simulink model "F104_Project_NEw_Aero_final_replacing"  (R2013a)
settings: Solver=ode45  StartTime=0.0  StopTime=50  FixedStep=0.01  RelTol=0.01
values from neighbouring files (symbols this model uses):
  b_w = 21.94    [Donee.m]
  C = 9.55    [Donee.m]
  Cl_beta = -0.09    [CX.m]    (also in CY.m; CZ.m; Cm.m; Cn.m)
  Cl_delta_aileron = 0.017    [Donee.m]
  CL_delta_elevator = 0.52    [Donee.m]
  Cl_delta_rudder = 0.008    [Donee.m]
  Cm_alpha = CL_alpha*CmoCL    [Aerodynamic_Dervatives.m]
  Cm_alpha_dot = - CL_alpha_dot * (l_t/C)    [Aerodynamic_Dervatives.m]
  Cm_delta_elevator = -0.2    [Donee.m]
  Cm_q = - CL_q * (l_t/C)    [Aerodynamic_Dervatives.m]
  Cm_u = 0    [Aerodynamic_Dervatives.m]
  Cn_beta = 0.0024    [Aerodynamic_Dervatives.m]    (also in CX.m = 0.24; CY.m = 0.24; CZ.m = 0.24; Cm.m = 0.24)
  Cn_delta_aileron = 0.0025    [Donee.m]
  Cn_delta_rudder = -0.04    [Donee.m]
  CX_q = -CD_q    (= 0)    [Aerodynamic_Dervatives.m]
  Cy_delta_rudder = 0.05    [Donee.m]
  CZ_alpha_dot = - CL_alpha_dot    [Aerodynamic_Dervatives.m]
  CZ_q = -CL_q    [Aerodynamic_Dervatives.m]
  S_w = (Cr_w + Ct_w)*b_w/4    (= 95.762615)    [Donee.m]
undefined symbols (not defined in the file or in its folder): Cl_beta_dot, Cl_p, Cl_r, Cn_beta_dot, Cn_p, Cn_r, CX_alpha, CX_u, Cy_beta, Cy_beta_dot, Cy_r, CZ_alpha, CZ_u, ft, kg, lbm, m, s
libraries: aerolibconvert2 x6, aerolibasang x2, aerolib6dof2 x1, aerolibatmos2 x1
settings Model: Creator=Ibrahim_B92  LastModifiedBy=Ibrahim_B92

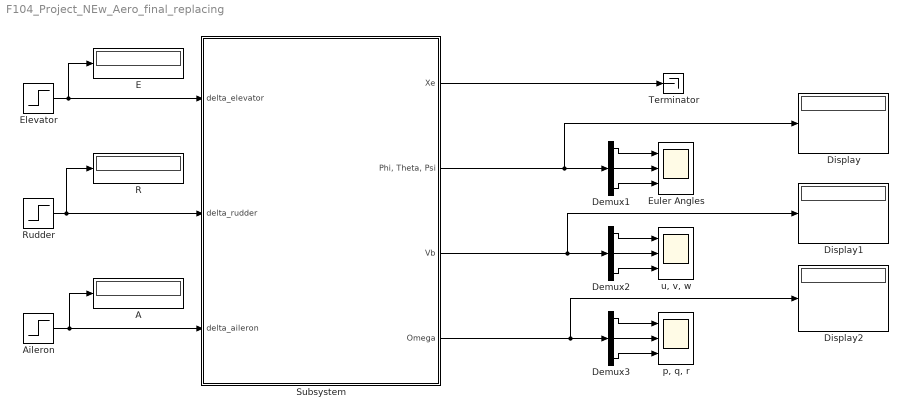
== system F104_Project_NEw_Aero_final_replacing ==
  A : Display
  Aileron : Step  Time=0  After=0  SampleTime=0
  Demux1 : Demux  Outputs=3
  Demux2 : Demux  Outputs=3
  Demux3 : Demux  Outputs=3
  Display : Display
  Display1 : Display
  Display2 : Display
  E : Display
  Elevator : Step  Time=0  After=0  SampleTime=0
  Euler Angles : Scope  NumInputPorts=3
      settings: TimeRange=16  YMin=0~-2~-5  YMax=1000~2~10
  R : Display
  Rudder : Step  Time=0  After=0  SampleTime=0
  Subsystem : Subsystem
  Terminator : Terminator
  "p, q, r" : Scope  NumInputPorts=3
      settings: TimeRange=10  YMin=-5~-5~-5  YMax=5~5~5  SaveName=ScopeData3
  "u, v, w" : Scope  NumInputPorts=3
      settings: TickLabels=on  TimeRange=16  YMin=-1000~-2000~-2000  YMax=2000~2000~2000  SaveName=ScopeData2
  wires:
  Subsystem/1(Xe) -> Terminator/1
  Demux1/1 -> Euler Angles/1
  Demux1/2 -> Euler Angles/2
  Demux1/3 -> Euler Angles/3
  Subsystem/2("Phi, Theta, Psi") -> Display/1, Demux1/1
  Demux2/1 -> "u, v, w"/1
  Demux2/2 -> "u, v, w"/2
  Demux2/3 -> "u, v, w"/3
  Subsystem/3(Vb) -> Display1/1, Demux2/1
  Demux3/1 -> "p, q, r"/1
  Demux3/2 -> "p, q, r"/2
  Demux3/3 -> "p, q, r"/3
  Subsystem/4(Omega) -> Display2/1, Demux3/1
  Rudder/1 -> Subsystem/2(delta_rudder), R/1
  Aileron/1 -> Subsystem/3(delta_aileron), A/1
  Elevator/1 -> Subsystem/1(delta_elevator), E/1

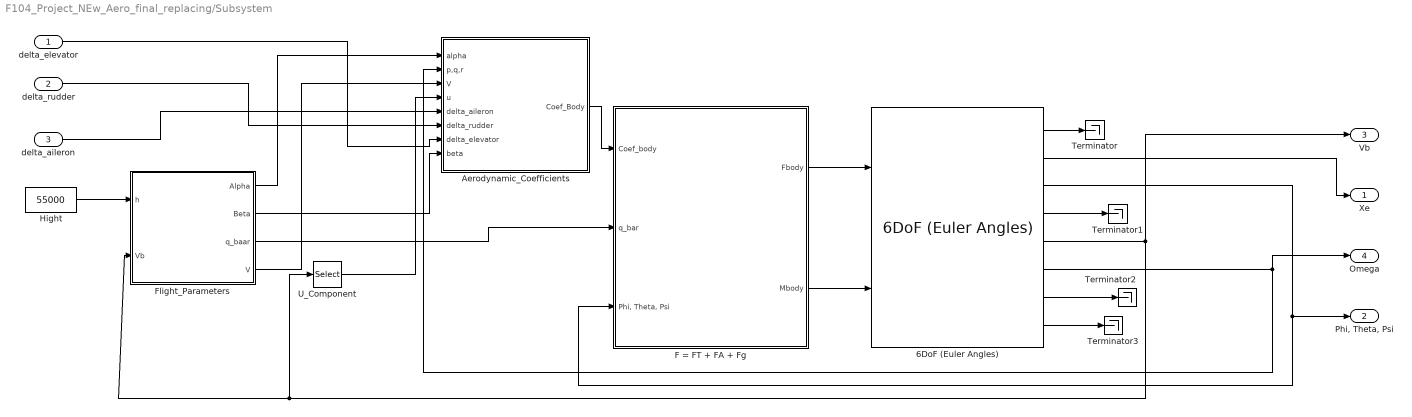
== system F104_Project_NEw_Aero_final_replacing/Subsystem ==
  delta_elevator : Inport
  delta_rudder : Inport  Port=2
  delta_aileron : Inport  Port=3
  6DoF (Euler Angles) : aerolib6dof2/6DoF (Euler Angles)  units=Metric (MKS)  mtype=Fixed  rep=Euler Angles  xme_0=|  Vm_0=|  eul_0=[0 0 0]  pm_0=[0 0 0]  mass_0=16300  mass_e=0.5  mass_f=2.0  inertia=Q  inertia_e=eye(3)  inertia_f=2*eye(3)  k_quat=1.0
      xme_0=|
      | [0
      | 0
      | -55000]
      Vm_0=|
      | [968*1.8
      | 0
      | 0]
  Aerodynamic_Coefficients : Subsystem
  F = FT + FA + Fg : Subsystem
  Flight_Parameters : Subsystem
  Hight : Constant  Value=55000
  Terminator{,1..3} (4 alike) : Terminator
  U_Component : Selector  InputPortWidth=3  IndexOptions=Index vector (dialog)  Indices=[1]  OutputSizes=1
  Xe : Outport
  "Phi, Theta, Psi" : Outport  Port=2
  Vb : Outport  Port=3
  Omega : Outport  Port=4
  wires:
  6DoF (Euler Angles)/2 -> Xe/1
  6DoF (Euler Angles)/3 -> F = FT + FA + Fg/3("Phi, Theta, Psi"), "Phi, Theta, Psi"/1
  6DoF (Euler Angles)/5 -> Flight_Parameters/2(Vb), U_Component/1, Vb/1
  6DoF (Euler Angles)/6 -> Aerodynamic_Coefficients/2(p,q,r), Omega/1
  F = FT + FA + Fg/1(Fbody) -> 6DoF (Euler Angles)/1
  F = FT + FA + Fg/2(Mbody) -> 6DoF (Euler Angles)/2
  Flight_Parameters/3(q_baar) -> F = FT + FA + Fg/2(q_bar)
  Flight_Parameters/1(Alpha) -> Aerodynamic_Coefficients/1(alpha)
  Flight_Parameters/2(Beta) -> Aerodynamic_Coefficients/8(beta)
  Hight/1 -> Flight_Parameters/1(h)
  Flight_Parameters/4(V) -> Aerodynamic_Coefficients/3(V)
  delta_elevator/1 -> Aerodynamic_Coefficients/7(delta_elevator)
  delta_rudder/1 -> Aerodynamic_Coefficients/6(delta_rudder)
  6DoF (Euler Angles)/1 -> Terminator/1
  6DoF (Euler Angles)/4 -> Terminator1/1
  6DoF (Euler Angles)/7 -> Terminator2/1
  6DoF (Euler Angles)/8 -> Terminator3/1
  U_Component/1 -> Aerodynamic_Coefficients/4(u)
  Aerodynamic_Coefficients/1(Coef_Body) -> F = FT + FA + Fg/1(Coef_body)
  delta_aileron/1 -> Aerodynamic_Coefficients/5(delta_aileron)

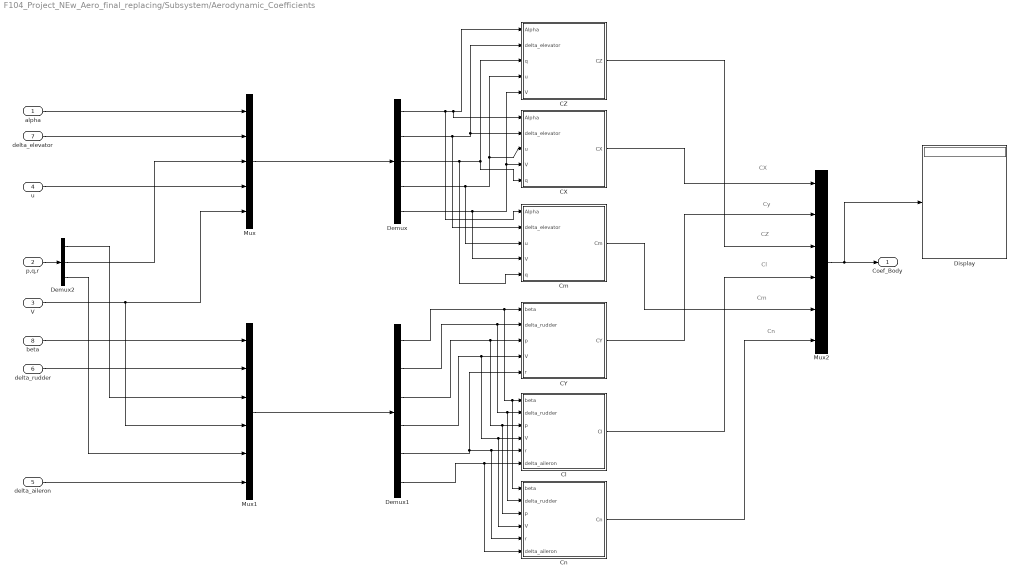
== system F104_Project_NEw_Aero_final_replacing/Subsystem/Aerodynamic_Coefficients ==
  note: Cn
  note: Cm
  note: Cl
  note: CZ
  note: Cy
  note: CX
  alpha : Inport
  p,q,r : Inport  Port=2
  V : Inport  Port=3
  u : Inport  Port=4
  delta_aileron : Inport  Port=5
  delta_rudder : Inport  Port=6
  delta_elevator : Inport  Port=7
  beta : Inport  Port=8
  CX : Subsystem
  CY : Subsystem
  CZ : Subsystem
  Cl : Subsystem
  Cm : Subsystem
  Cn : Subsystem
  Demux : Demux  Outputs=5
  Demux1 : Demux  Outputs=6
  Demux2 : Demux  Outputs=3
  Display : Display
  Mux : Mux  Inputs=5
  Mux1 : Mux  Inputs=6
  Mux2 : Mux  Inputs=6
  Coef_Body : Outport
  wires:
  Demux/1 -> Cm/1(Alpha), CX/1(Alpha), CZ/1(Alpha)
  Demux/2 -> Cm/2(delta_elevator), CX/2(delta_elevator), CZ/2(delta_elevator)
  Demux/3 -> Cm/5(q), CZ/3(q), CX/5(q)
  Demux/5 -> Cm/4(V), CX/4(V), CZ/5(V)
  Demux/4 -> Cm/3(u), CX/3(u), CZ/4(u)
  Demux1/1 -> Cn/1(beta), Cl/1(beta), CY/1(beta)
  Demux1/2 -> Cn/2(delta_rudder), Cl/2(delta_rudder), CY/2(delta_rudder)
  Demux1/4 -> Cn/4(V), Cl/4(V), CY/4(V)
  Demux1/5 -> CY/5(r), Cl/5(r), Cn/5(r)
  Demux1/6 -> Cn/6(delta_aileron), Cl/6(delta_aileron)
  Demux1/3 -> Cl/3(p), Cn/3(p), CY/3(p)
  Mux/1 -> Demux/1
  alpha/1 -> Mux/1
  p,q,r/1 -> Demux2/1
  delta_elevator/1 -> Mux/2
  Demux2/2 -> Mux/3
  u/1 -> Mux/4
  V/1 -> Mux1/4, Mux/5
  Mux1/1 -> Demux1/1
  beta/1 -> Mux1/1
  delta_rudder/1 -> Mux1/2
  Demux2/1 -> Mux1/3
  Demux2/3 -> Mux1/5
  delta_aileron/1 -> Mux1/6
  CX/1(CX) -> Mux2/1
  CY/1(CY) -> Mux2/2
  CZ/1(CZ) -> Mux2/3
  Cl/1(Cl) -> Mux2/4
  Cm/1(Cm) -> Mux2/5
  Cn/1(Cn) -> Mux2/6
  Mux2/1 -> Display/1, Coef_Body/1

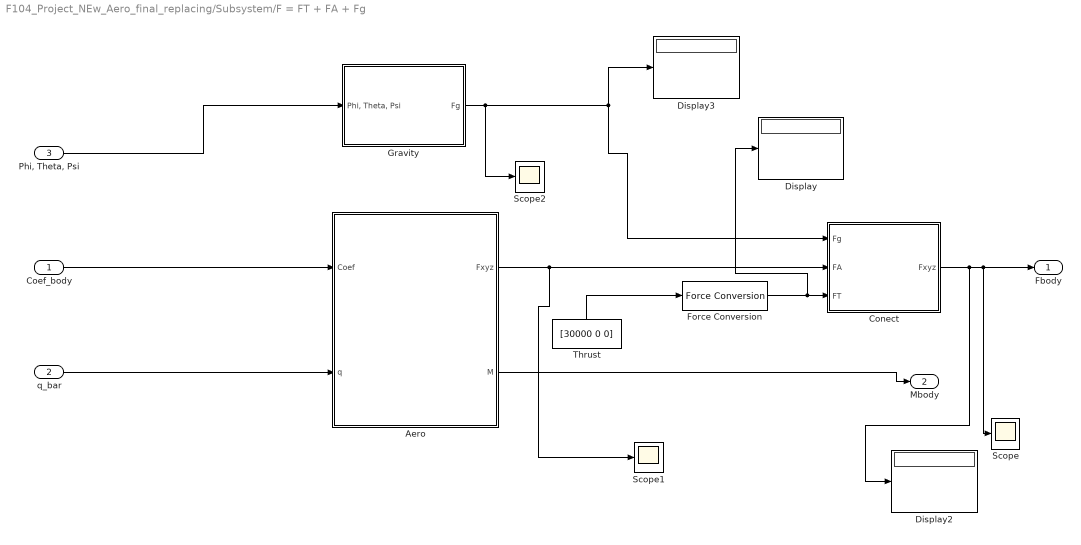
== system F104_Project_NEw_Aero_final_replacing/Subsystem/F = FT + FA + Fg ==
  Coef_body : Inport
  q_bar : Inport  Port=2
  "Phi, Theta, Psi" : Inport  Port=3
  "Aero " : Subsystem
  "Conect " : Subsystem
  Display : Display
  Display2 : Display
  Display3 : Display
  Force Conversion : aerolibconvert2/Force Conversion  IU=N  OU=lbf
  Gravity : Subsystem
  Scope : Scope
      settings: SaveName=ScopeData5
  Scope1 : Scope
      settings: SaveName=ScopeData9
  Scope2 : Scope
      settings: SaveName=ScopeData7
  Thrust : Constant  Value=[30000 0 0]
  Fbody : Outport
  Mbody : Outport  Port=2
  wires:
  "Aero "/1(Fxyz) -> Scope1/1, "Conect "/2(FA)
  "Aero "/2(M) -> Mbody/1
  "Conect "/1(Fxyz) -> Display2/1, Scope/1, Fbody/1
  Thrust/1 -> Force Conversion/1
  q_bar/1 -> "Aero "/2(q)
  Coef_body/1 -> "Aero "/1(Coef)
  Force Conversion/1 -> Display/1, "Conect "/3(FT)
  "Phi, Theta, Psi"/1 -> Gravity/1("Phi, Theta, Psi")
  Gravity/1(Fg) -> Scope2/1, "Conect "/1(Fg), Display3/1

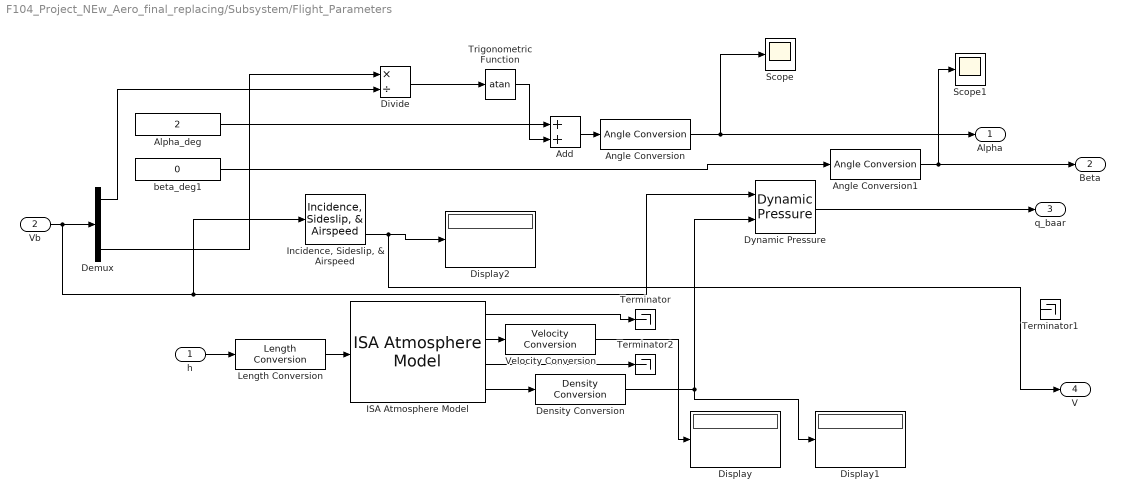
== system F104_Project_NEw_Aero_final_replacing/Subsystem/Flight_Parameters ==
  h : Inport
  Vb : Inport  Port=2
  Add : Sum
  Alpha_deg : Constant  Value=2
  Angle Conversion : aerolibconvert2/Angle Conversion  IU=deg  OU=rad
  Angle Conversion1 : aerolibconvert2/Angle Conversion  IU=deg  OU=rad
  Demux : Demux  Outputs=3
  Density Conversion : aerolibconvert2/Density Conversion  IU=kg/m^3  OU=lbm/ft^3
  Display : Display
  Display1 : Display
  Display2 : Display
  Divide : Product  Inputs=*/
  Dynamic Pressure : aerolibasang/Dynamic Pressure
  ISA Atmosphere Model : aerolibatmos2/ISA Atmosphere Model  custom=off  g=9.80665  gamma=1.4  R=287.0531  L=0.0065  h_trop=11000  h_strat=20000  rho0=1.225  P0=101325  T0=288.15  h0=0
  "Incidence, Sideslip, & Airspeed" : aerolibasang/Incidence, Sideslip, & Airspeed
  Length Conversion : aerolibconvert2/Length Conversion  IU=ft  OU=m
  Scope : Scope
  Scope1 : Scope
      settings: TimeRange=16  SaveName=ScopeData4
  Terminator : Terminator
  Terminator1 : Terminator
  Terminator2 : Terminator
  Trigonometric Function : Trigonometry  Operator=atan
  Velocity Conversion : aerolibconvert2/Velocity Conversion  IU=m/s  OU=ft/s
  beta_deg1 : Constant  Value=0
  Alpha : Outport
  Beta : Outport  Port=2
  q_baar : Outport  Port=3
  V : Outport  Port=4
  wires:
  h/1 -> Length Conversion/1
  Dynamic Pressure/1 -> q_baar/1
  ISA Atmosphere Model/4 -> Density Conversion/1
  ISA Atmosphere Model/1 -> Terminator/1
  ISA Atmosphere Model/2 -> Velocity Conversion/1
  ISA Atmosphere Model/3 -> Terminator2/1
  Density Conversion/1 -> Dynamic Pressure/2, Display1/1
  Velocity Conversion/1 -> Display/1
  Length Conversion/1 -> ISA Atmosphere Model/1
  Angle Conversion/1 -> Scope/1, Alpha/1
  Angle Conversion1/1 -> Scope1/1, Beta/1
  Vb/1 -> "Incidence, Sideslip, & Airspeed"/1, Dynamic Pressure/1, Demux/1
  Alpha_deg/1 -> Add/1
  Add/1 -> Angle Conversion/1
  beta_deg1/1 -> Angle Conversion1/1
  Demux/3 -> Divide/1
  Divide/1 -> Trigonometric Function/1
  Trigonometric Function/1 -> Add/2
  "Incidence, Sideslip, & Airspeed"/3 -> V/1, Display2/1
  Demux/1 -> Divide/2

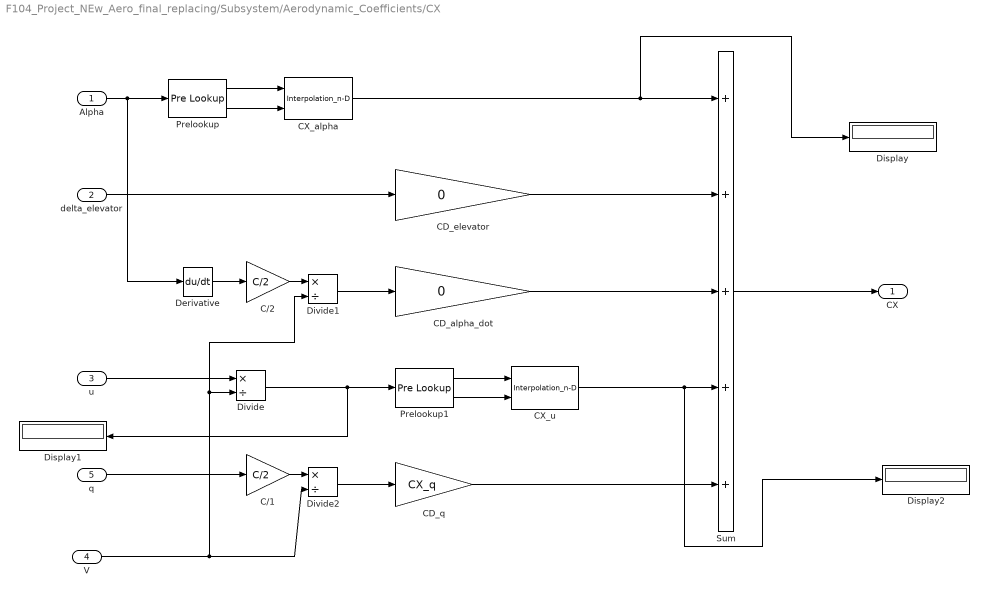
== system F104_Project_NEw_Aero_final_replacing/Subsystem/Aerodynamic_Coefficients/CX ==
  Alpha : Inport
  delta_elevator : Inport  Port=2
  u : Inport  Port=3
  V : Inport  Port=4
  q : Inport  Port=5
  C/1 : Gain  Gain=C/2
  C/2 : Gain  Gain=C/2
  CD_alpha_dot : Gain  Gain=0
  CD_elevator : Gain  Gain=0
  CD_q : Gain  Gain=CX_q
  CX_alpha : Interpolation_n-D  NumberOfTableDimensions=1  Table=CX_alpha
      settings: InputPortMap=u0,u1
  CX_u : Interpolation_n-D  NumberOfTableDimensions=1  Table=CX_u
      settings: InputPortMap=u0,u1
  Derivative : Derivative
  Display : Display
  Display1 : Display
  Display2 : Display
  Divide : Product  Inputs=*/
  Divide1 : Product  Inputs=*/
  Divide2 : Product  Inputs=*/
  Prelookup : PreLookup  BreakpointsData=alpha  ExtrapMethod=Linear
  Prelookup1 : PreLookup  BreakpointsData=alpha  ExtrapMethod=Linear
  Sum : Sum  Inputs=+++++
  CX : Outport
  wires:
  delta_elevator/1 -> CD_elevator/1
  u/1 -> Divide/1
  Divide/1 -> Display1/1, Prelookup1/1
  CX_alpha/1 -> Display/1, Sum/1
  CD_elevator/1 -> Sum/2
  CD_alpha_dot/1 -> Sum/3
  Sum/1 -> CX/1
  V/1 -> Divide1/2, Divide/2, Divide2/2
  Prelookup/1 -> CX_alpha/1
  Prelookup/2 -> CX_alpha/2
  C/2/1 -> Divide1/1
  Divide1/1 -> CD_alpha_dot/1
  Alpha/1 -> Derivative/1, Prelookup/1
  C/1/1 -> Divide2/1
  q/1 -> C/1/1
  Divide2/1 -> CD_q/1
  Prelookup1/1 -> CX_u/1
  Prelookup1/2 -> CX_u/2
  Derivative/1 -> C/2/1
  CD_q/1 -> Sum/5
  CX_u/1 -> Display2/1, Sum/4

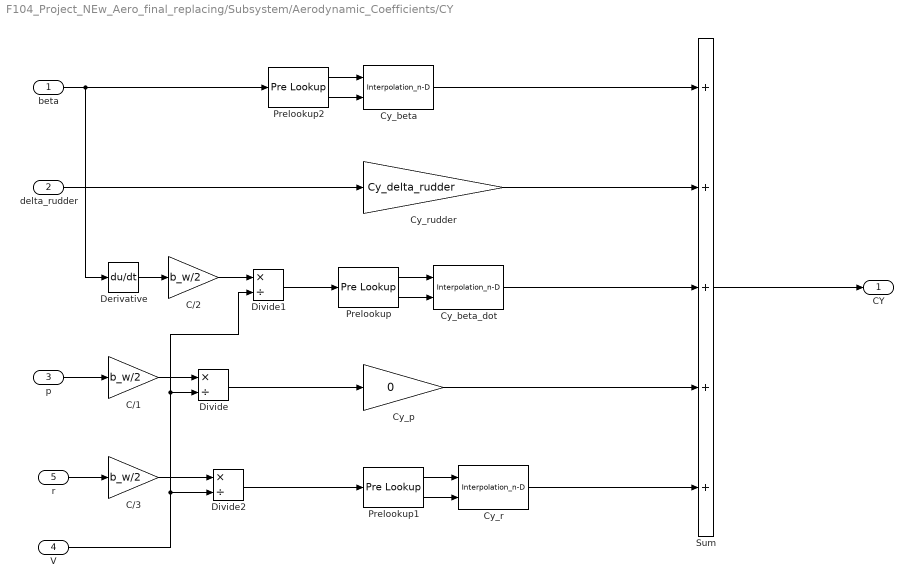
== system F104_Project_NEw_Aero_final_replacing/Subsystem/Aerodynamic_Coefficients/CY ==
  beta : Inport
  delta_rudder : Inport  Port=2
  p : Inport  Port=3
  V : Inport  Port=4
  r : Inport  Port=5
  C/1 : Gain  Gain=b_w/2
  C/2 : Gain  Gain=b_w/2
  C/3 : Gain  Gain=b_w/2
  Cy_beta : Interpolation_n-D  NumberOfTableDimensions=1  Table=Cy_beta
      settings: InputPortMap=u0,u1
  Cy_beta_dot : Interpolation_n-D  NumberOfTableDimensions=1  Table=Cy_beta_dot
      settings: InputPortMap=u0,u1
  Cy_p : Gain  Gain=0
  Cy_r : Interpolation_n-D  NumberOfTableDimensions=1  Table=Cy_r
      settings: InputPortMap=u0,u1
  Cy_rudder : Gain  Gain=Cy_delta_rudder
  Derivative : Derivative
  Divide : Product  Inputs=*/
  Divide1 : Product  Inputs=*/
  Divide2 : Product  Inputs=*/
  Prelookup : PreLookup  BreakpointsData=alpha  ExtrapMethod=Linear
  Prelookup1 : PreLookup  BreakpointsData=alpha  ExtrapMethod=Linear
  Prelookup2 : PreLookup  BreakpointsData=alpha  ExtrapMethod=Linear
  Sum : Sum  Inputs=+++++
  CY : Outport
  wires:
  delta_rudder/1 -> Cy_rudder/1
  beta/1 -> Prelookup2/1, Derivative/1
  p/1 -> C/1/1
  Divide/1 -> Cy_p/1
  r/1 -> C/3/1
  Cy_beta/1 -> Sum/1
  Cy_rudder/1 -> Sum/2
  Cy_beta_dot/1 -> Sum/3
  Cy_p/1 -> Sum/4
  Sum/1 -> CY/1
  V/1 -> Divide2/2, Divide1/2, Divide/2
  Prelookup/1 -> Cy_beta_dot/1
  Prelookup/2 -> Cy_beta_dot/2
  C/2/1 -> Divide1/1
  Divide1/1 -> Prelookup/1
  Derivative/1 -> C/2/1
  C/1/1 -> Divide/1
  Divide2/1 -> Prelookup1/1
  C/3/1 -> Divide2/1
  Prelookup1/1 -> Cy_r/1
  Prelookup1/2 -> Cy_r/2
  Cy_r/1 -> Sum/5
  Prelookup2/1 -> Cy_beta/1
  Prelookup2/2 -> Cy_beta/2

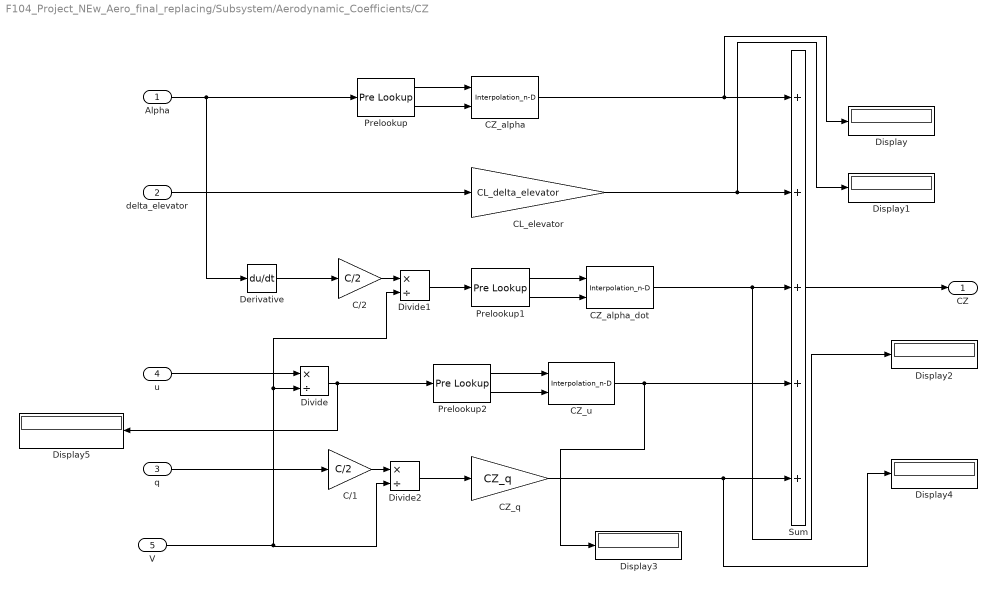
== system F104_Project_NEw_Aero_final_replacing/Subsystem/Aerodynamic_Coefficients/CZ ==
  Alpha : Inport
  delta_elevator : Inport  Port=2
  q : Inport  Port=3
  u : Inport  Port=4
  V : Inport  Port=5
  C/1 : Gain  Gain=C/2
  C/2 : Gain  Gain=C/2
  CL_elevator : Gain  Gain=CL_delta_elevator
  CZ_alpha : Interpolation_n-D  NumberOfTableDimensions=1  Table=CZ_alpha
      settings: InputPortMap=u0,u1
  CZ_alpha_dot : Interpolation_n-D  NumberOfTableDimensions=1  Table=CZ_alpha_dot
      settings: InputPortMap=u0,u1
  CZ_q : Gain  Gain=CZ_q
  CZ_u : Interpolation_n-D  NumberOfTableDimensions=1  Table=CZ_u
      settings: InputPortMap=u0,u1
  Derivative : Derivative
  Display{,1..5} (6 alike) : Display
  Divide : Product  Inputs=*/
  Divide1 : Product  Inputs=*/
  Divide2 : Product  Inputs=*/
  Prelookup : PreLookup  BreakpointsData=alpha  ExtrapMethod=Linear
  Prelookup1 : PreLookup  BreakpointsData=alpha  ExtrapMethod=Linear
  Prelookup2 : PreLookup  BreakpointsData=alpha  ExtrapMethod=Linear  DiagnosticForOutOfRangeInput=Warning
  Sum : Sum  Inputs=+++++
  CZ : Outport
  wires:
  delta_elevator/1 -> CL_elevator/1
  Alpha/1 -> Prelookup/1, Derivative/1
  CZ_alpha/1 -> Display/1, Sum/1
  CL_elevator/1 -> Display1/1, Sum/2
  CZ_alpha_dot/1 -> Display2/1, Sum/3
  Sum/1 -> CZ/1
  u/1 -> Divide/1
  V/1 -> Divide2/2, Divide/2, Divide1/2
  C/2/1 -> Divide1/1
  Divide1/1 -> Prelookup1/1
  Derivative/1 -> C/2/1
  C/1/1 -> Divide2/1
  Divide2/1 -> CZ_q/1
  q/1 -> C/1/1
  Prelookup/1 -> CZ_alpha/1
  Prelookup/2 -> CZ_alpha/2
  Prelookup1/1 -> CZ_alpha_dot/1
  Prelookup1/2 -> CZ_alpha_dot/2
  Prelookup2/2 -> CZ_u/2
  Prelookup2/1 -> CZ_u/1
  CZ_q/1 -> Display4/1, Sum/5
  CZ_u/1 -> Sum/4, Display3/1
  Divide/1 -> Prelookup2/1, Display5/1

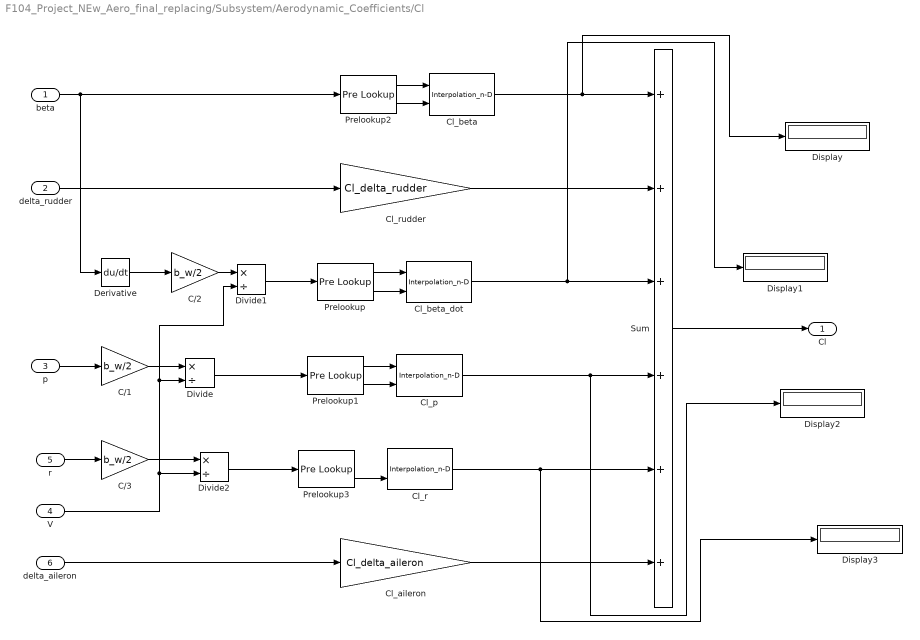
== system F104_Project_NEw_Aero_final_replacing/Subsystem/Aerodynamic_Coefficients/Cl ==
  beta : Inport
  delta_rudder : Inport  Port=2
  p : Inport  Port=3
  V : Inport  Port=4
  r : Inport  Port=5
  delta_aileron : Inport  Port=6
  C/1 : Gain  Gain=b_w/2
  C/2 : Gain  Gain=b_w/2
  C/3 : Gain  Gain=b_w/2
  Cl_aileron : Gain  Gain=Cl_delta_aileron
  Cl_beta : Interpolation_n-D  NumberOfTableDimensions=1  Table=Cl_beta
      settings: InputPortMap=u0,u1
  Cl_beta_dot : Interpolation_n-D  NumberOfTableDimensions=1  Table=Cl_beta_dot
      settings: InputPortMap=u0,u1
  Cl_p : Interpolation_n-D  NumberOfTableDimensions=1  Table=Cl_p
      settings: InputPortMap=u0,u1
  Cl_r : Interpolation_n-D  NumberOfTableDimensions=1  Table=Cl_r
      settings: InputPortMap=u0,u1
  Cl_rudder : Gain  Gain=Cl_delta_rudder
  Derivative : Derivative
  Display{,1..3} (4 alike) : Display
  Divide : Product  Inputs=*/
  Divide1 : Product  Inputs=*/
  Divide2 : Product  Inputs=*/
  Prelookup{,1..3} (4 alike) : PreLookup  BreakpointsData=alpha  ExtrapMethod=Linear
  Sum : Sum  Inputs=++++++
  Cl : Outport
  wires:
  delta_rudder/1 -> Cl_rudder/1
  beta/1 -> Prelookup2/1, Derivative/1
  p/1 -> C/1/1
  Divide/1 -> Prelookup1/1
  r/1 -> C/3/1
  Cl_beta/1 -> Display/1, Sum/1
  Cl_rudder/1 -> Sum/2
  Cl_beta_dot/1 -> Display1/1, Sum/3
  Cl_p/1 -> Display2/1, Sum/4
  Cl_r/1 -> Display3/1, Sum/5
  Sum/1 -> Cl/1
  V/1 -> Divide2/2, Divide1/2, Divide/2
  Prelookup/1 -> Cl_beta_dot/1
  Prelookup/2 -> Cl_beta_dot/2
  C/2/1 -> Divide1/1
  Divide1/1 -> Prelookup/1
  Derivative/1 -> C/2/1
  C/1/1 -> Divide/1
  Divide2/1 -> Prelookup3/1
  C/3/1 -> Divide2/1
  Prelookup1/1 -> Cl_p/1
  Prelookup1/2 -> Cl_p/2
  delta_aileron/1 -> Cl_aileron/1
  Cl_aileron/1 -> Sum/6
  Prelookup2/1 -> Cl_beta/1
  Prelookup2/2 -> Cl_beta/2
  Prelookup3/2 -> Cl_r/2

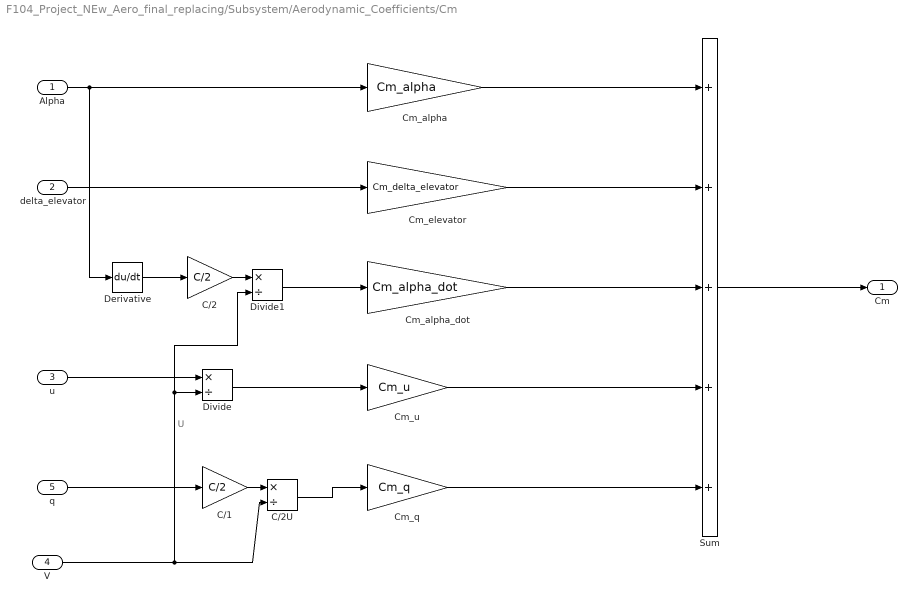
== system F104_Project_NEw_Aero_final_replacing/Subsystem/Aerodynamic_Coefficients/Cm ==
  note: U
  Alpha : Inport
  delta_elevator : Inport  Port=2
  u : Inport  Port=3
  V : Inport  Port=4
  q : Inport  Port=5
  C/1 : Gain  Gain=C/2
  C/2 : Gain  Gain=C/2
  C/2U : Product  Inputs=*/
  Cm_alpha : Gain  Gain=Cm_alpha
  Cm_alpha_dot : Gain  Gain=Cm_alpha_dot
  Cm_elevator : Gain  Gain=Cm_delta_elevator
  Cm_q : Gain  Gain=Cm_q
  Cm_u : Gain  Gain=Cm_u
  Derivative : Derivative
  Divide : Product  Inputs=*/
  Divide1 : Product  Inputs=*/
  Sum : Sum  Inputs=+++++
  Cm : Outport
  wires:
  delta_elevator/1 -> Cm_elevator/1
  Alpha/1 -> Derivative/1, Cm_alpha/1
  u/1 -> Divide/1
  Divide/1 -> Cm_u/1
  Cm_alpha/1 -> Sum/1
  Cm_elevator/1 -> Sum/2
  Cm_alpha_dot/1 -> Sum/3
  Cm_u/1 -> Sum/4
  Cm_q/1 -> Sum/5
  Sum/1 -> Cm/1
  C/2/1 -> Divide1/1
  Divide1/1 -> Cm_alpha_dot/1
  C/1/1 -> C/2U/1
  q/1 -> C/1/1
  C/2U/1 -> Cm_q/1
  V/1 -> Divide/2, Divide1/2, C/2U/2
  Derivative/1 -> C/2/1

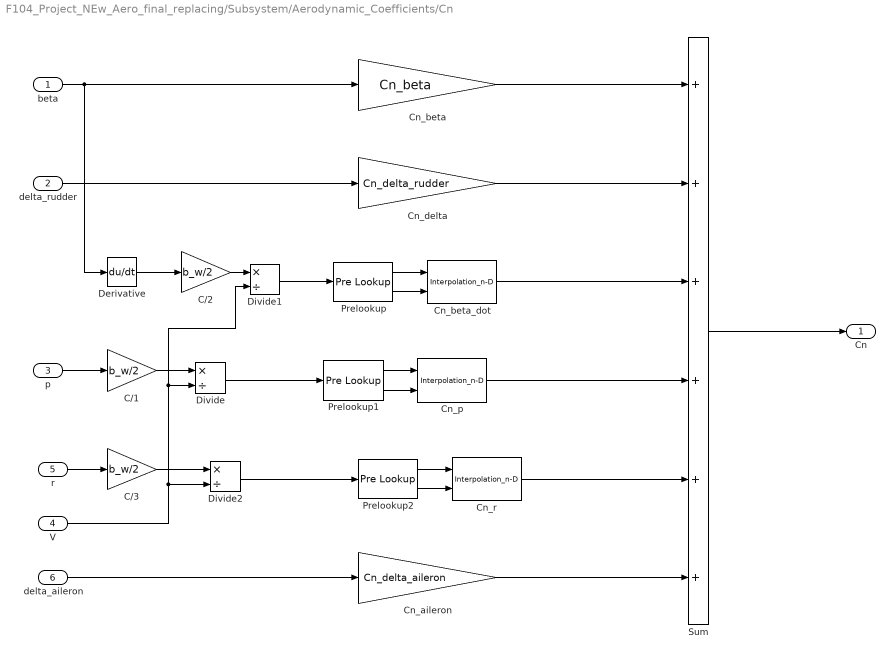
== system F104_Project_NEw_Aero_final_replacing/Subsystem/Aerodynamic_Coefficients/Cn ==
  beta : Inport
  delta_rudder : Inport  Port=2
  p : Inport  Port=3
  V : Inport  Port=4
  r : Inport  Port=5
  delta_aileron : Inport  Port=6
  C/1 : Gain  Gain=b_w/2
  C/2 : Gain  Gain=b_w/2
  C/3 : Gain  Gain=b_w/2
  Cn_aileron : Gain  Gain=Cn_delta_aileron
  Cn_beta : Gain  Gain=Cn_beta
  Cn_beta_dot : Interpolation_n-D  NumberOfTableDimensions=1  Table=Cn_beta_dot
      settings: InputPortMap=u0,u1
  Cn_delta : Gain  Gain=Cn_delta_rudder
  Cn_p : Interpolation_n-D  NumberOfTableDimensions=1  Table=Cn_p
      settings: InputPortMap=u0,u1
  Cn_r : Interpolation_n-D  NumberOfTableDimensions=1  Table=Cn_r
      settings: InputPortMap=u0,u1
  Derivative : Derivative
  Divide : Product  Inputs=*/
  Divide1 : Product  Inputs=*/
  Divide2 : Product  Inputs=*/
  Prelookup : PreLookup  BreakpointsData=alpha  ExtrapMethod=Linear
  Prelookup1 : PreLookup  BreakpointsData=alpha  ExtrapMethod=Linear
  Prelookup2 : PreLookup  BreakpointsData=alpha  ExtrapMethod=Linear
  Sum : Sum  Inputs=++++++
  Cn : Outport
  wires:
  delta_rudder/1 -> Cn_delta/1
  beta/1 -> Cn_beta/1, Derivative/1
  p/1 -> C/1/1
  Divide/1 -> Prelookup1/1
  r/1 -> C/3/1
  Cn_beta/1 -> Sum/1
  Cn_delta/1 -> Sum/2
  Cn_beta_dot/1 -> Sum/3
  Cn_p/1 -> Sum/4
  Cn_r/1 -> Sum/5
  Sum/1 -> Cn/1
  V/1 -> Divide2/2, Divide1/2, Divide/2
  Prelookup/1 -> Cn_beta_dot/1
  Prelookup/2 -> Cn_beta_dot/2
  C/2/1 -> Divide1/1
  Divide1/1 -> Prelookup/1
  Derivative/1 -> C/2/1
  C/1/1 -> Divide/1
  Divide2/1 -> Prelookup2/1
  C/3/1 -> Divide2/1
  Prelookup1/1 -> Cn_p/1
  Prelookup1/2 -> Cn_p/2
  delta_aileron/1 -> Cn_aileron/1
  Cn_aileron/1 -> Sum/6
  Prelookup2/2 -> Cn_r/2
  Prelookup2/1 -> Cn_r/1

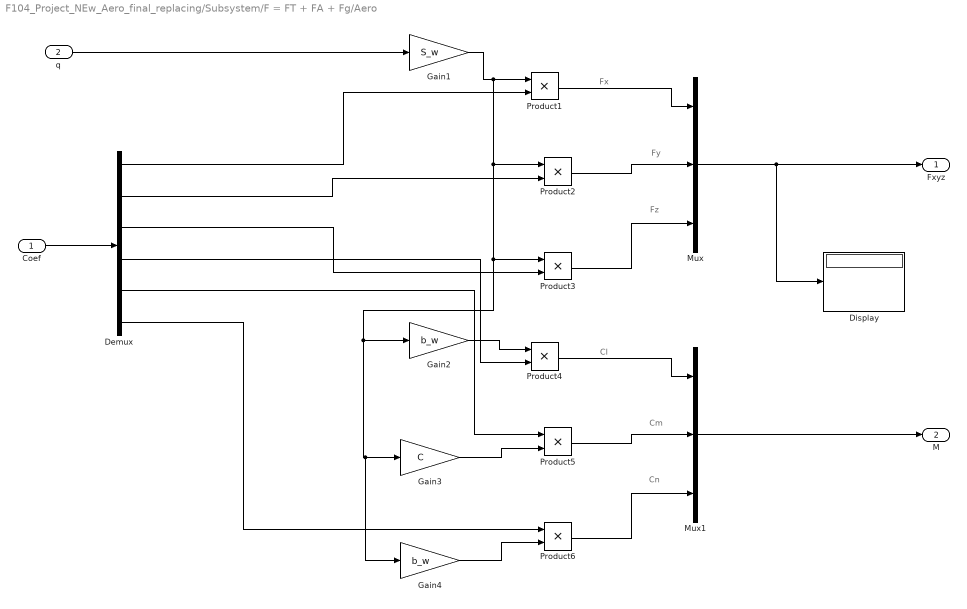
== system F104_Project_NEw_Aero_final_replacing/Subsystem/F = FT + FA + Fg/Aero  ==
  note: Fz
  note: Fy
  note: Fx
  note: Cn
  note: Cm
  note: Cl
  Coef : Inport
  q : Inport  Port=2
  Demux : Demux  Outputs=6
  Display : Display
  Gain1 : Gain  Gain=S_w
  Gain2 : Gain  Gain=b_w
  Gain3 : Gain  Gain=C
  Gain4 : Gain  Gain=b_w
  Mux : Mux  Inputs=3
  Mux1 : Mux  Inputs=3
  Product{1..6} (6 alike) : Product
  Fxyz : Outport
  M : Outport  Port=2
  wires:
  Coef/1 -> Demux/1
  Demux/1 -> Product1/2
  Gain1/1 -> Gain4/1, Gain3/1, Gain2/1, Product3/1, Product2/1, Product1/1
  Product1/1 -> Mux/1
  Demux/2 -> Product2/2
  Product2/1 -> Mux/2
  Demux/3 -> Product3/2
  Product3/1 -> Mux/3
  Product4/1 -> Mux1/1
  Product5/1 -> Mux1/2
  Product6/1 -> Mux1/3
  Gain2/1 -> Product4/1
  Demux/4 -> Product4/2
  Gain3/1 -> Product5/2
  Demux/5 -> Product5/1
  Gain4/1 -> Product6/2
  Demux/6 -> Product6/1
  Mux1/1 -> M/1
  Mux/1 -> Display/1, Fxyz/1
  q/1 -> Gain1/1

== system F104_Project_NEw_Aero_final_replacing/Subsystem/F = FT + FA + Fg/Conect  ==
  Fg : Inport
  FA : Inport  Port=2
  FT : Inport  Port=3
  Demux : Demux  Outputs=3
  Demux1 : Demux  Outputs=3
  Demux2 : Demux  Outputs=3
  Mux : Mux  Inputs=3
  Sum : Sum  Inputs=+++
  Sum1 : Sum  Inputs=+++
  Sum2 : Sum  Inputs=+++
  Fxyz : Outport
  wires:
  Fg/1 -> Demux/1
  FA/1 -> Demux1/1
  FT/1 -> Demux2/1
  Demux/1 -> Sum/1
  Demux1/1 -> Sum/2
  Demux2/1 -> Sum/3
  Demux/2 -> Sum1/1
  Demux1/2 -> Sum1/2
  Demux2/2 -> Sum1/3
  Demux/3 -> Sum2/1
  Demux1/3 -> Sum2/2
  Demux2/3 -> Sum2/3
  Sum/1 -> Mux/1
  Mux/1 -> Fxyz/1
  Sum1/1 -> Mux/2
  Sum2/1 -> Mux/3

== system F104_Project_NEw_Aero_final_replacing/Subsystem/F = FT + FA + Fg/Gravity ==
  note: Psi
  note: Theta
  note: Phi
  "Phi, Theta, Psi" : Inport
  Demux : Demux  Outputs=3
  Gravity Acceleration : Gain  Gain=32.174
  Mass : Gain  Gain=16300
  Mux : Mux  Inputs=3
  Product : Product
  Product1 : Product
  Scope : Scope
      settings: SaveName=ScopeData6
  T : Trigonometry
  T1 : Trigonometry
  T2 : Trigonometry  Operator=cos
  T3 : Trigonometry  Operator=cos
  T4 : Trigonometry  Operator=cos
  Terminator : Terminator
  Fg : Outport
  wires:
  T3/1 -> Product1/1
  T4/1 -> Product1/2
  T1/1 -> Product/1
  T2/1 -> Product/2
  "Phi, Theta, Psi"/1 -> Demux/1
  Demux/2 -> T4/1, T2/1, T/1
  Demux/1 -> T3/1, T1/1
  Demux/3 -> Terminator/1
  T/1 -> Mux/1
  Product/1 -> Mux/2
  Product1/1 -> Mux/3
  Mux/1 -> Mass/1
  Mass/1 -> Gravity Acceleration/1
  Gravity Acceleration/1 -> Scope/1, Fg/1
